simulink model "task_3"  (R2023b)
settings: Solver=FixedStepAuto  StartTime=0.0  StopTime=1000  FixedStep=1e-3  RelTol=1e-3
values from neighbouring files (symbols this model uses):
  A = [0, 1; -a0 -a1] + [0 0; 20 20]    [task_2.m]    (also in task_3.m)
  A_M = [0 1; -a_M0 -a_M1]    [task_2.m]    (also in task_3.m)
  b = [0; b0]    [task_2.m]    (also in task_3.m)
  b_M = [0; a_M0]    [task_2.m]    (also in task_3.m)
  C = eye(2)    [task_2.m]    (also in task_3.m)
  g = 1    [task_3.m]
  gamma = 100    [task_3.m]
  kappa = b0/a_M0    (= 0.074549499703)    [task_2.m]    (also in task_3.m)
  P = lyap(A_M', Q)    [task_3.m]
  theta = [theta1; theta2]    [task_2.m]    (also in task_3.m)
settings Model: Creator=nguye  LastModifiedBy=nguye

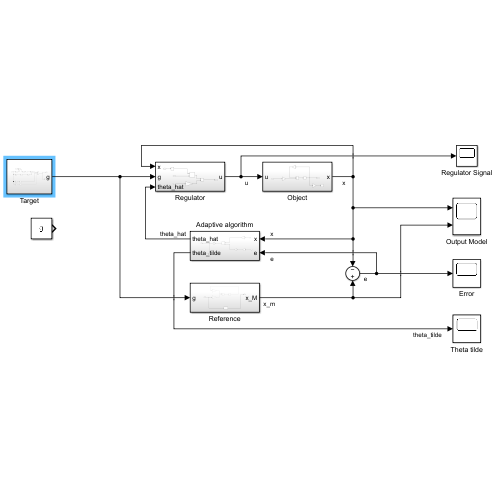
[thumbnail: Simulink's stored preview of the top-level diagram]
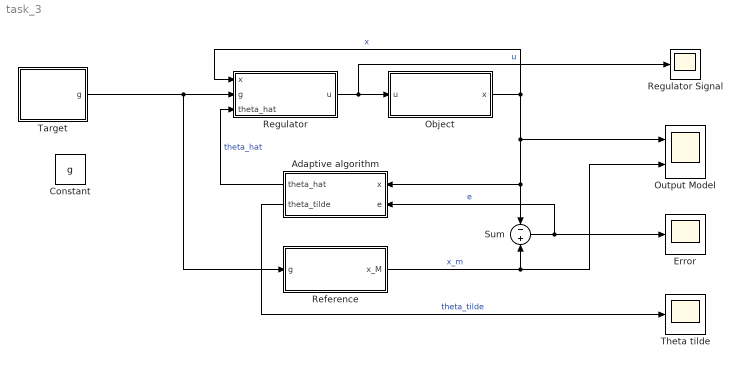
== system task_3 ==
  Adaptive algorithm : Subsystem
  Constant : Constant  Value=g
  Error : Scope
  Object : Subsystem
  Output Model : Scope  NumInputPorts=2
  Reference : Subsystem
  Regulator : Subsystem
  Regulator Signal : Scope
  Sum : Sum  Inputs=-|+
  Target : Subsystem
  Theta tilde : Scope
  wires:
  Regulator/1(u) -> Regulator Signal/1, Object/1(u)  "u"
  Object/1(x) -> Regulator/1(x), Output Model/1, Sum/1, Adaptive algorithm/1(x)  "x"
  Adaptive algorithm/1(theta_hat) -> Regulator/3(theta_hat)  "theta_hat"
  Reference/1(x_M) -> Sum/2, Output Model/2  "x_m"
  Sum/1 -> Error/1, Adaptive algorithm/2(e)  "e"
  Adaptive algorithm/2(theta_tilde) -> Theta tilde/1  "theta_tilde"
  Target/1(g) -> Reference/1(g), Regulator/2(g)

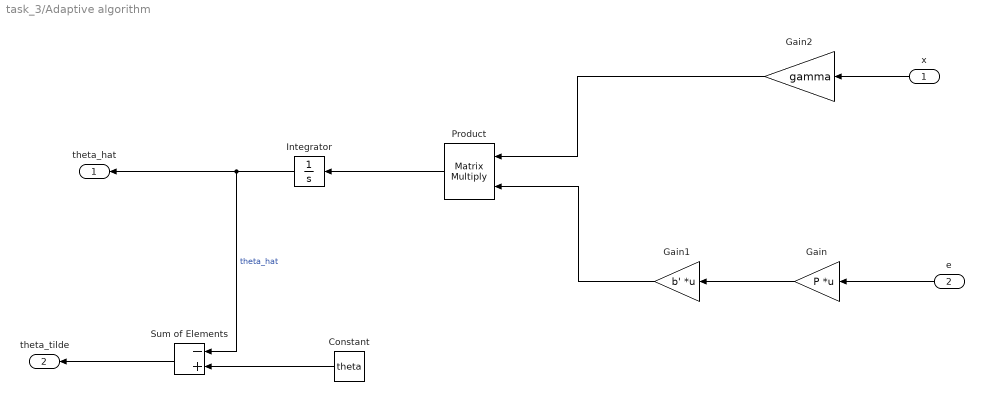
== system task_3/Adaptive algorithm ==
  x : Inport
  e : Inport  Port=2
  Constant : Constant  Value=theta
  Gain : Gain  Gain=P  Multiplication=Matrix(K*u)
  Gain1 : Gain  Gain=b'  Multiplication=Matrix(K*u)
  Gain2 : Gain  Gain=gamma
  Integrator : Integrator
  Product : Product  Multiplication=Matrix(*)
  Sum of Elements : Sum  Inputs=-+
  theta_hat : Outport
  theta_tilde : Outport  Port=2
  wires:
  Integrator/1 -> Sum of Elements/1, theta_hat/1  "theta_hat"
  e/1 -> Gain/1
  Gain/1 -> Gain1/1
  x/1 -> Gain2/1
  Gain1/1 -> Product/2
  Gain2/1 -> Product/1
  Product/1 -> Integrator/1
  Sum of Elements/1 -> theta_tilde/1
  Constant/1 -> Sum of Elements/2

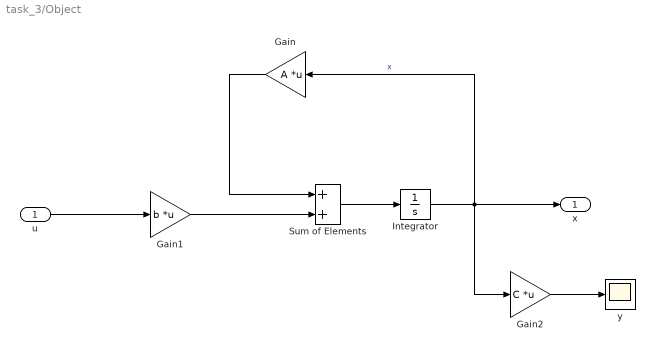
== system task_3/Object ==
  u : Inport
  Gain : Gain  Gain=A  Multiplication=Matrix(K*u)
  Gain1 : Gain  Gain=b  Multiplication=Matrix(K*u)
  Gain2 : Gain  Gain=C  Multiplication=Matrix(K*u)
  Integrator : Integrator  InitialCondition=1
  Sum of Elements : Sum
  y : Scope
  x : Outport
  wires:
  Sum of Elements/1 -> Integrator/1
  Gain/1 -> Sum of Elements/1
  Gain1/1 -> Sum of Elements/2
  u/1 -> Gain1/1
  Integrator/1 -> Gain/1, Gain2/1, x/1  "x"
  Gain2/1 -> y/1

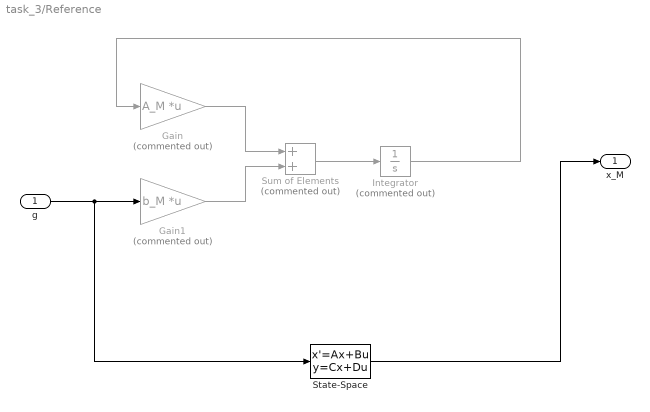
== system task_3/Reference ==
  g : Inport
  Gain : Gain  Commented=on  Gain=A_M  Multiplication=Matrix(K*u)
  Gain1 : Gain  Commented=on  Gain=b_M  Multiplication=Matrix(K*u)
  Integrator : Integrator  Commented=on  InitialCondition=[0;0]
  State-Space : StateSpace  A=A_M  B=b_M  C=eye(2)  D=zeros(2,1)  InitialCondition=0
  Sum of Elements : Sum  Commented=on
  x_M : Outport
  wires:
  g/1 -> State-Space/1, Gain1/1
  Gain1/1 -> Sum of Elements/2
  Gain/1 -> Sum of Elements/1
  Sum of Elements/1 -> Integrator/1
  Integrator/1 -> Gain/1
  State-Space/1 -> x_M/1

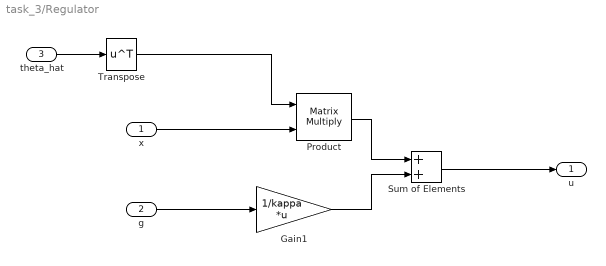
== system task_3/Regulator ==
  x : Inport
  g : Inport  Port=2
  theta_hat : Inport  Port=3
  Gain1 : Gain  Gain=1/kappa  Multiplication=Matrix(K*u)
  Product : Product  Multiplication=Matrix(*)
  Sum of Elements : Sum
  Transpose : Math  Operator=transpose
  u : Outport
  wires:
  x/1 -> Product/2
  Product/1 -> Sum of Elements/1
  Gain1/1 -> Sum of Elements/2
  g/1 -> Gain1/1
  Sum of Elements/1 -> u/1
  theta_hat/1 -> Transpose/1
  Transpose/1 -> Product/1

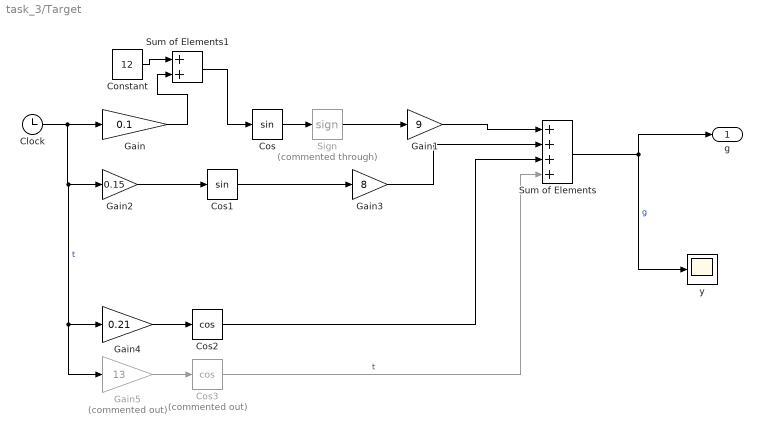
== system task_3/Target ==
  Clock : Clock
  Constant : Constant  Value=12
  Cos : Trigonometry
  Cos1 : Trigonometry
  Cos2 : Trigonometry  Operator=cos
  Cos3 : Trigonometry  Commented=on  Operator=cos
  Gain : Gain  Gain=0.1
  Gain1 : Gain  Gain=9
  Gain2 : Gain  Gain=0.15
  Gain3 : Gain  Gain=8
  Gain4 : Gain  Gain=0.21
  Gain5 : Gain  Commented=on  Gain=13
  Sign : Signum  Commented=through
  Sum of Elements : Sum  Inputs=++++
  Sum of Elements1 : Sum
  y : Scope
  g : Outport
  wires:
  Clock/1 -> Gain5/1, Gain4/1, Gain2/1, Gain/1  "t"
  Cos/1 -> Sign/1
  Cos2/1 -> Sum of Elements/3
  Sum of Elements/1 -> g/1, y/1  "g"
  Gain/1 -> Sum of Elements1/2
  Gain1/1 -> Sum of Elements/1
  Cos1/1 -> Gain3/1
  Gain3/1 -> Sum of Elements/2
  Gain2/1 -> Cos1/1
  Gain4/1 -> Cos2/1
  Sign/1 -> Gain1/1
  Gain5/1 -> Cos3/1
  Cos3/1 -> Sum of Elements/4  "t"
  Constant/1 -> Sum of Elements1/1
  Sum of Elements1/1 -> Cos/1
